simulink model "abenics_pid_plant"  (R2026a)
settings: Solver=ode4  StopTime=10  FixedStep=pp.Ts_plant
PreLoadFcn:
  | params_abenics;
undefined symbols (not defined in the file or in its folder): pp
libraries: slpidlib x1
settings Model: Creator=aminaik  LastModifiedBy=aminaik

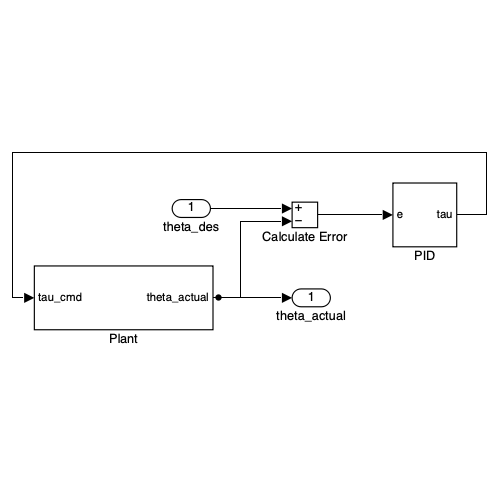
[thumbnail: Simulink's stored preview of the top-level diagram]
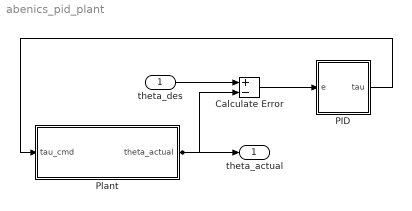
== system abenics_pid_plant ==
  theta_des : Inport  PortDimensions=4
  Calculate Error : Sum  Inputs=+-
  PID : Subsystem
  Plant : Subsystem
  theta_actual : Outport  PortDimensions=4
  wires:
  PID/1(tau) -> Plant/1(tau_cmd)
  Calculate Error/1 -> PID/1(e)
  Plant/1(theta_actual) -> Calculate Error/2, theta_actual/1
  theta_des/1 -> Calculate Error/1

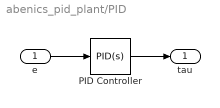
== system abenics_pid_plant/PID ==
  e : Inport
  PID Controller : slpidlib/PID Controller  Controller=PID  Form=Parallel  TimeDomain=Continuous-time  UseExternalTs=off  SampleTime=-1  IntegratorMethod=Forward Euler  FilterMethod=Forward Euler  ControllerParametersSource=internal  P=pp.Kp  I=pp.Ki  UseKiTs=off  D=pp.Kd  UseExternalDerivativeSource=off  N=pp.N  UseFilter=on  TunerSelectOption=Transfer Function Based (PID Tuner App)  InitialConditionSource=internal  InitialConditionForIntegrator=0  InitialConditionForFilter=0  DifferentiatorICPrevScaledInput=0  ExternalReset=none  TrackingMode=off  Kt=1  LimitOutput=on  SatLimitsSource=internal  UpperSaturationLimit=pp.tau_max  LowerSaturationLimit=-pp.tau_max  LinearizeAsGain=on  AntiWindupMode=clamping  Kb=1  LimitIntegrator=off  UpperIntegratorSaturationLimit=inf  LowerIntegratorSaturationLimit=-inf  POutMin=[]  POutMax=[]  IOutMin=[]  IOutMax=[]  DOutMin=[]  DOutMax=[]  NOutMin=[]  NOutMax=[]  SumOutMin=[]  SumOutMax=[]  SaturationOutMin=[]  SaturationOutMax=[]  PParamMin=[]  PParamMax=[]  IParamMin=[]  IParamMax=[]  DParamMin=[]  DParamMax=[]  NParamMin=[]  NParamMax=[]  KbParamMin=[]  KbParamMax=[]  KtParamMin=[]  KtParamMax=[]  KbOutMin=[]  KbOutMax=[]  KtOutMin=[]  KtOutMax=[]  IntegratorOutMin=[]  IntegratorOutMax=[]  FilterOutMin=[]  FilterOutMax=[]  SumI1OutMin=[]  SumI1OutMax=[]  SumI2OutMin=[]  SumI2OutMax=[]  SumI3OutMin=[]  SumI3OutMax=[]  SumI4OutMin=[]  SumI4OutMax=[]  SumDOutMin=[]  SumDOutMax=[]  DifferentiatorOutMin=[]  DifferentiatorOutMax=[]  FilterDiffOutCoefMin=[]  FilterDiffOutCoefMax=[]  ReciprocalOutMin=[]  ReciprocalOutMax=[]  SumDenOutMin=[]  SumDenOutMax=[]  SumNumOutMin=[]  SumNumOutMax=[]  DivideOutMin=[]  DivideOutMax=[]  UdiffTsProdOutMin=[]  UdiffTsProdOutMax=[]  NTsProdOutMin=[]  NTsProdOutMax=[]  UintegralTsProdOutMin=[]  UintegralTsProdOutMax=[]  UngainTsProdOutMin=[]  UngainTsProdOutMax=[]  ClampingZeroOutDataTypeStr=Inherit: Inherit via back propagation  ClampingZeroOutMin=[]  ClampingZeroOutMax=[]  FilterDenConstantOutDataTypeStr=Inherit: Inherit via back propagation  FilterDenConstantOutMin=[]  FilterDenConstantOutMax=[]  PCopyOutDataTypeStr=Inherit: Inherit via back propagation  PCopyOutMin=[]  PCopyOutMax=[]  NCopyOutDataTypeStr=Inherit: Inherit via back propagation  NCopyOutMin=[]  NCopyOutMax=[]  IntegratorContinuousStateAttributes=''  IntegratorStateMustResolveToSignalObject=off  IntegratorRTWStateStorageClass=Auto  FilterContinuousStateAttributes=''  FilterStateMustResolveToSignalObject=off  FilterRTWStateStorageClass=Auto  ParallelPVariant=InternalParameters  IdealPVariant=Disabled  IVariant=InternalParameters  DVariant=InternalParameters  IntegratorVariant=Continuous  SatVariant=Enabled  AWVariant=ContClampingParallel  PCopyVariant=Disabled  TRVariant=Disabled  FdbkBlocksVariant=Forward  IdealPFdbkVariant=Disabled  SatFdbkVariant=Disabled  DerivativeFilterVariant=ContFilter  NVariant=InternalParameters  NCopyVariant=Disabled  FilterICVariant=InternalICsFilter  IntegratorICVariant=InternalICs  ExternalResetVariant=Disabled  TRSumVariant=Passthrough  SumFdbkVariant=Disabled  SumVariant=Sum_PID  TsampFilterVariant=InternalTs  TsampNgainVariant=Passthrough  TsampIntegralVariant=Disabled_SignalSpec  ExternalSaturationOutDataTypeStr=Inherit: Same as second input  DerivativeSourceVariant=ErrorSignal  PreIntVariant=InternalPreInt
  tau : Outport
  wires:
  PID Controller/1 -> tau/1
  e/1 -> PID Controller/1

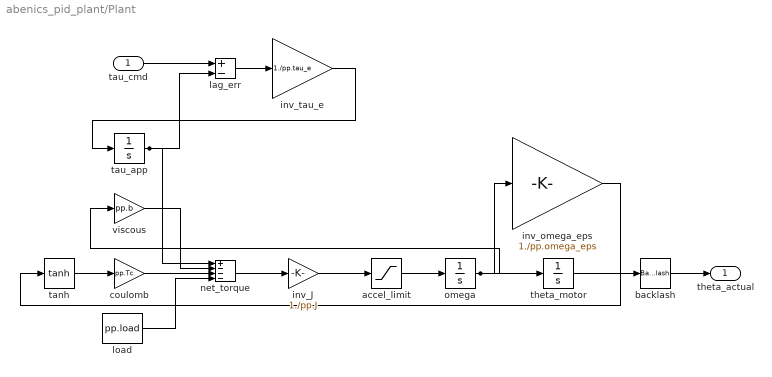
== system abenics_pid_plant/Plant ==
  tau_cmd : Inport
  accel_limit : Saturate  UpperLimit=pp.alpha_max  LowerLimit=-pp.alpha_max
  backlash : Backlash  BacklashWidth=pp.backlash  InitialOutput=pp.theta0
  coulomb : Gain  Gain=pp.Tc
  inv_J : Gain  Gain=1./pp.J
  inv_omega_eps : Gain  Gain=1./pp.omega_eps
  inv_tau_e : Gain  Gain=1./pp.tau_e
  lag_err : Sum  Inputs=+-
  load : Constant  Value=pp.load
  net_torque : Sum  Inputs=+---
  omega : Integrator  InitialCondition=pp.omega0  LimitOutput=on  UpperSaturationLimit=pp.omega_max  LowerSaturationLimit=-pp.omega_max
  tanh : Trigonometry  Operator=tanh
  tau_app : Integrator
  theta_motor : Integrator  InitialCondition=pp.theta0
  viscous : Gain  Gain=pp.b
  theta_actual : Outport
  wires:
  inv_omega_eps/1 -> tanh/1
  omega/1 -> inv_omega_eps/1, theta_motor/1, viscous/1
  inv_J/1 -> accel_limit/1
  theta_motor/1 -> backlash/1
  inv_tau_e/1 -> tau_app/1
  accel_limit/1 -> omega/1
  lag_err/1 -> inv_tau_e/1
  load/1 -> net_torque/4
  coulomb/1 -> net_torque/3
  backlash/1 -> theta_actual/1
  net_torque/1 -> inv_J/1
  tau_app/1 -> net_torque/1, lag_err/2
  viscous/1 -> net_torque/2
  tau_cmd/1 -> lag_err/1
  tanh/1 -> coulomb/1
